simulink model "sensorExpoler_Lab_11"  (R2026a)
settings: Solver=FixedStepDiscrete  StopTime=inf  FixedStep=0.001
undefined symbols (not defined in the file): Blocking, Non
libraries: amg_usbconverter_n_connect_lib x2
settings Model: Creator=pboon  LastModifiedBy=Lenovo

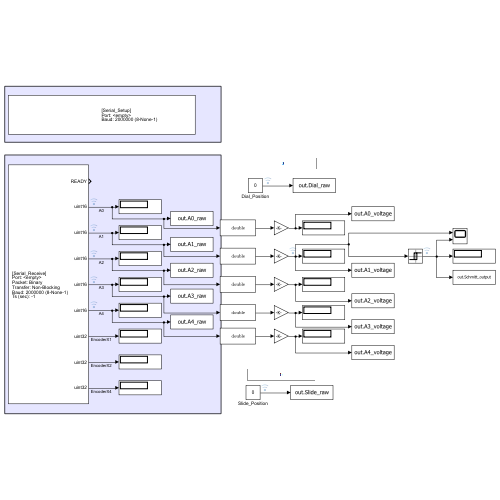
[thumbnail: Simulink's stored preview of the top-level diagram]
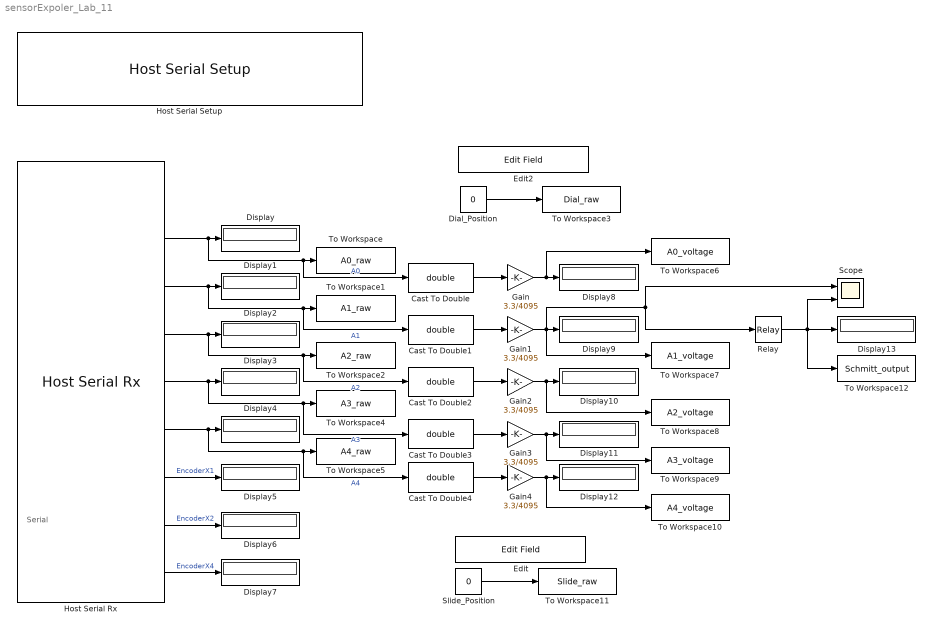
== system sensorExpoler_Lab_11 ==
  note: Serial
  Cast To Double{,1..4} (5 alike) : DataTypeConversion  OutDataTypeStr=double  SaturateOnIntegerOverflow=off  RndMeth=Floor
  Dial_Position : Constant  Value=0  OutDataTypeStr=double  SampleTime=0.001
  Display{,1..13} (14 alike) : Display
  Edit : EditField  LabelPosition=Hide  ShowInitialText=on  Alignment=Center
  Edit2 : EditField  LabelPosition=Hide  ShowInitialText=on  Alignment=Center
  Gain{,1..4} (5 alike) : Gain  Gain=3.3/4095
  Host Serial Rx : amg_usbconverter_n_connect_lib/Host Serial Rx  conf=rx  port=<auto>  baudrate=2000000  databits=8  parity=None  stopbit=1  flowcontrol=None  transfer=Non-Blocking  timeout=5  packetmode=Binary  enableinitialvalues=off  initialvalues=[]  binheader='25'  binterminator='4E 4E'  porttype_double=0  porttype_single=0  porttype_int8=0  porttype_uint8=0  porttype_int16=0  porttype_uint16=5  porttype_int32=0  porttype_uint32=3  asciiformat='%d,%f'  rx_asciiterminator="CRLF (0x0D 0x0A - \"\\r\\n\")"  tx_asciiterminator="CRLF (0x0D 0x0A - \"\\r\\n\")"  sampletime=0.001  enablecustomportlabel=off  cinputportlabel=0  coutputportlabel=A  portpinstr=0  blockid=HostSerialRx  inputporttype=[]  inputportwidth=[]  inputportlabel={}  outputporttype=[3 5 5 5 5 5 7 7 7]  outputportwidth=[1 1 1 1 1 1 1 1 1]  outputportlabel={'READY','uint16','uint16','uint16','uint16','uint16','uint32','uint32','uint32'}  compat=0  optionstring=[]  autoport='<empty>'
  Host Serial Setup : amg_usbconverter_n_connect_lib/Host Serial Setup  conf=setup  port=<auto>  baudrate=2000000  databits=8  parity=None  stopbit=1  flowcontrol=None  transfer=Blocking  timeout=2  packetmode=Binary  initialvalues=[]  binheader='7E 7E'  binterminator='03 03'  porttype_double=0  porttype_single=1  porttype_int8=0  porttype_uint8=0  porttype_int16=0  porttype_uint16=0  porttype_int32=0  porttype_uint32=2  asciiformat='%d %u %x'  rx_asciiterminator="CRLF (0x0D 0x0A - \"\\r\\n\")"  tx_asciiterminator="CRLF (0x0D 0x0A - \"\\r\\n\")"  sampletime=-1  enablecustomportlabel=off  cinputportlabel=0  coutputportlabel=A  portpinstr=0  blockid=HostSerialSetup  inputporttype=[]  inputportwidth=[]  inputportlabel={}  outputporttype=[]  outputportwidth=[]  outputportlabel={}  compat=0  optionstring=[]  autoport='<empty>'
  Relay : Relay  OnSwitchValue=2.0  OffSwitchValue=1.0
  Scope : Scope  NumInputPorts=2
      settings: ActiveDisplayYMinimum=0.17930981626619102  ActiveDisplayYMaximum=1.8678303234536924
  Slide_Position : Constant  Value=0
  To Workspace : ToWorkspace  VariableName=A0_raw  SaveFormat=Timeseries  SampleTime=-1
  To Workspace1 : ToWorkspace  VariableName=A1_raw  SaveFormat=Timeseries  SampleTime=-1
  To Workspace10 : ToWorkspace  VariableName=A4_voltage  SaveFormat=Timeseries  SampleTime=-1
  To Workspace11 : ToWorkspace  VariableName=Slide_raw  SaveFormat=Timeseries  SampleTime=-1
  To Workspace12 : ToWorkspace  VariableName=Schmitt_output  SaveFormat=Timeseries  SampleTime=-1
  To Workspace2 : ToWorkspace  VariableName=A2_raw  SaveFormat=Timeseries  SampleTime=-1
  To Workspace3 : ToWorkspace  VariableName=Dial_raw  SaveFormat=Timeseries  SampleTime=-1
  To Workspace4 : ToWorkspace  VariableName=A3_raw  SaveFormat=Timeseries  SampleTime=-1
  To Workspace5 : ToWorkspace  VariableName=A4_raw  SaveFormat=Timeseries  SampleTime=-1
  To Workspace6 : ToWorkspace  VariableName=A0_voltage  SaveFormat=Timeseries  SampleTime=-1
  To Workspace7 : ToWorkspace  VariableName=A1_voltage  SaveFormat=Timeseries  SampleTime=-1
  To Workspace8 : ToWorkspace  VariableName=A2_voltage  SaveFormat=Timeseries  SampleTime=-1
  To Workspace9 : ToWorkspace  VariableName=A3_voltage  SaveFormat=Timeseries  SampleTime=-1
  wires:
  Host Serial Rx/2 -> Cast To Double/1, To Workspace/1, Display/1  "A0"
  Host Serial Rx/3 -> Cast To Double1/1, To Workspace1/1, Display1/1  "A1"
  Host Serial Rx/4 -> Cast To Double2/1, To Workspace2/1, Display2/1  "A2"
  Host Serial Rx/5 -> Cast To Double3/1, To Workspace4/1, Display3/1  "A3"
  Host Serial Rx/6 -> Cast To Double4/1, To Workspace5/1, Display4/1  "A4"
  Host Serial Rx/7 -> Display5/1  "EncoderX1"
  Host Serial Rx/8 -> Display6/1  "EncoderX2"
  Host Serial Rx/9 -> Display7/1  "EncoderX4"
  Dial_Position/1 -> To Workspace3/1
  Cast To Double/1 -> Gain/1
  Cast To Double1/1 -> Gain1/1
  Cast To Double2/1 -> Gain2/1
  Cast To Double3/1 -> Gain3/1
  Cast To Double4/1 -> Gain4/1
  Gain/1 -> To Workspace6/1, Display8/1
  Gain1/1 -> Scope/1, Relay/1, Display9/1, To Workspace7/1
  Gain2/1 -> To Workspace8/1, Display10/1
  Gain3/1 -> To Workspace9/1, Display11/1
  Gain4/1 -> To Workspace10/1, Display12/1
  Slide_Position/1 -> To Workspace11/1
  Relay/1 -> Scope/2, Display13/1, To Workspace12/1
